simulink model "Controller"  (R2025a)
settings: Solver=ode45  StartTime=0.0  StopTime=100  RelTol=1e-5
PreLoadFcn:
  | [aircraft, state] = astSkyHogg();
undefined symbols (not defined in the file): aircraft, getCoefficient, state
libraries: aerolibasang x3, slpidlib x2, aerolibfltsims x2, shared3dof x1, sharedtransform x1
settings Model: Creator=Likith  LastModifiedBy=Likith
settings SolverCC: AlgebraicLoopSolver=TrustRegion  MinimalZcImpactIntegration=on  MaxZcPerStep=1.0
settings DataIOCC: SaveFormat=Array
settings OptimizationCC: EnhancedBackFolding=on  StrengthReduction=on  InitFltsAndDblsToZero=on  DifferentSizesBufferReuse=on
settings DebuggingCC: WriteAfterWriteMsg=DisableAll  AlgebraicLoopMsg=none  FcnCallInpInsideContextMsg=warning  UniqueDataStoreMsg=error  RootOutportRequireBusObject=none  StateNameClashWarn=warning  StrictBusMsg=ErrorOnBusTreatedAsVector  SFUnexpectedBacktrackingDiag=warning  SFNoUnconditionalDefaultTransitionDiag=warning  SFExecutionAtInitializationDiag=none  ArithmeticOperatorsInVariantConditions=warning
settings ModelReferenceCC: EnableRefExpFcnMdlSchedulingChecks=on  PropagateSignalLabelsOutOfModel=off
settings SFSimCC: SimUseLocalCustomCode=off
settings RTWCC: RTWUseLocalCustomCode=off  GPUComputeCapability=3.5  DLArmComputeVersion=19.05
settings CodeAppCC: StateflowObjectComments=on

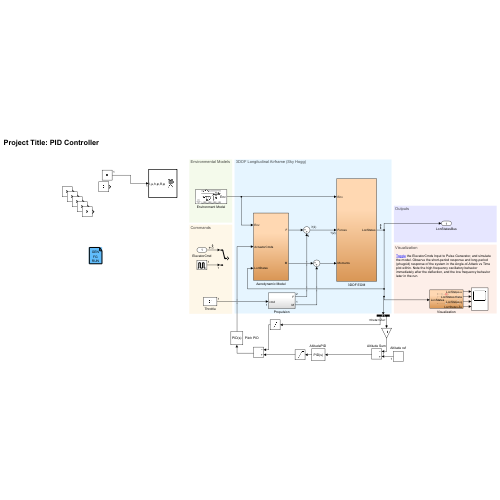
[thumbnail: Simulink's stored preview of the top-level diagram]
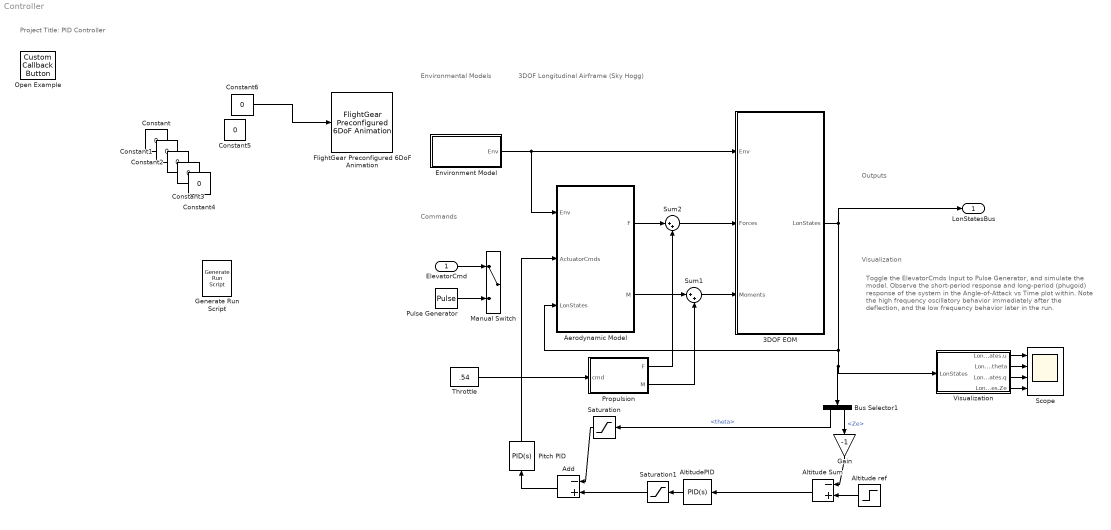
== system Controller ==
  note: Project Title: PID Controller
  note: 3DOF Longitudinal Airframe (Sky Hogg)
  note: Environmental Models
  note: Commands
  note: Toggle the ElevatorCmds Input to Pulse Generator, and simulate the model. Observe the short-period response and long-period (phugoid) response of the system in the Angle-of-Attack vs Time plot within. Note the high frequency oscillatory behavior immediately after the deflection, and the low frequency behavior later in the run.
  note: Visualization
  note: Outputs
  ElevatorCmd : Inport
  3DOF EOM : Subsystem  VariantControl=eom3DOF
  Add : Sum  Inputs=-+
  Aerodynamic Model : Subsystem  VariantControl=aeroCONST
  Altitude Sum : Sum  Inputs=-+
  Altitude ref : Step  Time=5  Before=2000  After=2200  SampleTime=0
  "AltitudePID " : slpidlib/PID Controller  Controller=PID  Form=Parallel  TimeDomain=Continuous-time  UseExternalTs=off  SampleTime=-1  IntegratorMethod=Forward Euler  FilterMethod=Forward Euler  ControllerParametersSource=internal  P=.05  I=.005  UseKiTs=off  D=0  UseExternalDerivativeSource=off  N=100  UseFilter=on  TunerSelectOption=Transfer Function Based (PID Tuner App)  InitialConditionSource=internal  InitialConditionForIntegrator=0  InitialConditionForFilter=0  DifferentiatorICPrevScaledInput=0  ExternalReset=none  TrackingMode=off  Kt=1  LimitOutput=off  SatLimitsSource=internal  UpperSaturationLimit=inf  LowerSaturationLimit=-inf  LinearizeAsGain=on  AntiWindupMode=none  Kb=1  LimitIntegrator=off  UpperIntegratorSaturationLimit=inf  LowerIntegratorSaturationLimit=-inf  POutMin=[]  POutMax=[]  IOutMin=[]  IOutMax=[]  DOutMin=[]  DOutMax=[]  NOutMin=[]  NOutMax=[]  SumOutMin=[]  SumOutMax=[]  SaturationOutMin=[]  SaturationOutMax=[]  PParamMin=[]  PParamMax=[]  IParamMin=[]  IParamMax=[]  DParamMin=[]  DParamMax=[]  NParamMin=[]  NParamMax=[]  KbParamMin=[]  KbParamMax=[]  KtParamMin=[]  KtParamMax=[]  KbOutMin=[]  KbOutMax=[]  KtOutMin=[]  KtOutMax=[]  IntegratorOutMin=[]  IntegratorOutMax=[]  FilterOutMin=[]  FilterOutMax=[]  SumI1OutMin=[]  SumI1OutMax=[]  SumI2OutMin=[]  SumI2OutMax=[]  SumI3OutMin=[]  SumI3OutMax=[]  SumI4OutMin=[]  SumI4OutMax=[]  SumDOutMin=[]  SumDOutMax=[]  DifferentiatorOutMin=[]  DifferentiatorOutMax=[]  FilterDiffOutCoefMin=[]  FilterDiffOutCoefMax=[]  ReciprocalOutMin=[]  ReciprocalOutMax=[]  SumDenOutMin=[]  SumDenOutMax=[]  SumNumOutMin=[]  SumNumOutMax=[]  DivideOutMin=[]  DivideOutMax=[]  UdiffTsProdOutMin=[]  UdiffTsProdOutMax=[]  NTsProdOutMin=[]  NTsProdOutMax=[]  UintegralTsProdOutMin=[]  UintegralTsProdOutMax=[]  UngainTsProdOutMin=[]  UngainTsProdOutMax=[]  ClampingZeroOutDataTypeStr=Inherit: Inherit via back propagation  ClampingZeroOutMin=[]  ClampingZeroOutMax=[]  FilterDenConstantOutDataTypeStr=Inherit: Inherit via back propagation  FilterDenConstantOutMin=[]  FilterDenConstantOutMax=[]  PCopyOutDataTypeStr=Inherit: Inherit via back propagation  PCopyOutMin=[]  PCopyOutMax=[]  NCopyOutDataTypeStr=Inherit: Inherit via back propagation  NCopyOutMin=[]  NCopyOutMax=[]  IntegratorContinuousStateAttributes=''  IntegratorStateMustResolveToSignalObject=off  IntegratorRTWStateStorageClass=Auto  FilterContinuousStateAttributes=''  FilterStateMustResolveToSignalObject=off  FilterRTWStateStorageClass=Auto  ParallelPVariant=InternalParameters  IdealPVariant=Disabled  IVariant=InternalParameters  DVariant=InternalParameters  IntegratorVariant=Continuous  SatVariant=Disabled  AWVariant=Passthrough  PCopyVariant=Disabled  TRVariant=Disabled  FdbkBlocksVariant=Forward  IdealPFdbkVariant=Disabled  SatFdbkVariant=Disabled  DerivativeFilterVariant=ContFilter  NVariant=InternalParameters  NCopyVariant=Disabled  FilterICVariant=InternalICsFilter  IntegratorICVariant=InternalICs  ExternalResetVariant=Disabled  TRSumVariant=Passthrough  SumFdbkVariant=Disabled  SumVariant=Sum_PID  TsampFilterVariant=InternalTs  TsampNgainVariant=Passthrough  TsampIntegralVariant=Disabled_SignalSpec  ExternalSaturationOutDataTypeStr=Inherit: Same as second input  DerivativeSourceVariant=ErrorSignal  PreIntVariant=InternalPreInt
  Bus Selector1 : BusSelector  OutputSignals=theta,Ze
  Constant{,1..6} (7 alike) : Constant  Value=0
  Environment Model : Subsystem  mask(Constant Environment Model){To=state.Environment.Temperature, a=state.Environment.SpeedOfSound, Po=state.Environment.Pressure, AirDensity=state.Environment.Density, ugvgwg=state.Environment.WindVelocity, pgqgrg=[0,0,0], g=[0;0;state.Environment.Gravity]}
      mask prompts: To "Constant Temperature (K):"; a "Constant Speed of Sound (m/s):"; Po "Constant Pressure (Pa):"; AirDensity "Constant Air Density (kg/m^3):"; ugvgwg "Constant Wind Velocity [ug vg wg] (m/s):"; pgqgrg "Constant Wind Angular Rates [pg qg rg] (rad/s):"; g "Constant Gravitational Acceleration (m/s^2):"
      mask Help: helpview(fullfile(docroot,'toolbox','aeroblks','aeroblks.map'), 'environment1');
      mask TypeOptions To: Constant Atmosphere/To
      mask TypeOptions a: Constant Atmosphere/a
      mask TypeOptions Po: Constant Atmosphere/Po
      mask TypeOptions AirDensity: Constant Atmosphere/AirDensity
      mask TypeOptions ugvgwg: Constant Wind/ugvgwg
      mask TypeOptions pgqgrg: Constant Wind/pgqgrg
      mask TypeOptions g: Constant Gravity/g
      mask DialogControl Container4 Prompt: Atmospheric Model
      mask DialogControl Container6 Prompt: Wind Model
      mask DialogControl Container8 Prompt: Gravity Model
      mask Display:
      | image('aeroenvironment.bmp','center')
      | port_label('output',1,'Env')
  FlightGear Preconfigured 6DoF Animation : aerolibfltsims/FlightGear Preconfigured 6DoF Animation  xFlightGearVersion=v2019.1  DestinationIpAddress=127.0.0.1  DestinationPort=5502  SampleTime=1/30  packetVersion=24
  Gain : Gain  Gain=-1
  Generate Run Script : aerolibfltsims/Generate Run Script  Architecture=Default  dataFlow=Send  GeometryModelName=HL20  AirportId=KSFO  RunwayId=10L  InitialAltitude=7224  InitialHeading=113  OffsetDistance=4.72  OffsetAzimuth=0  InstallScenery=off  DisableShaders=off  OriginAddress=127.0.0.1  DestinationPort=5502  OriginPort=5505  LocalAddress=127.0.0.1  OutputFileName=runfg.bat  FlightGearBaseDirectory=C:\Program Files\FlightGear
  Manual Switch : ManualSwitch
  Open Example : CustomCallbackButton  Configuration="{\"components\":[{\"name\":\"BackgroundImageComponent\",\"settings\":{\"image\":{\"size\":[0,0],\"src\":\"default\",\"srcOrientation\":\"Right\"},\"position\":[0,0,1,1]}},{\"name\":\"ButtonStateComponent\",\"settings\":{\"buttonType\":\"momentary\",\"clickFcn\":\"showExample('aeroblks\\/LongitudinalFlyingQuality3DOFAnalysisExample')\",\"onValue\":1,\"position\":[0,0,1,1],\"pressDelay\":\"500\",\"pressFcn\":\"\",\"repeatInterval\":\"0\",\"states\":[{\"horizontalAlignment\":\"center\",\"image\":{\"position\":[0,0,1,1],\"size\":[1,1],\"src\":\"default\",\"srcOrientation\":\"Right\"},\"label\":{\"color\":[0.01176470588,0.01176470588,0.01176470588,1],\"icon\":{\"size\":[0,0],\"src\":\"default\",\"srcOrientation\":\"Right\"},\"iconPlacement\":\"left\",\"opacity\":1,\"show\":true,\"text\":{\"content\":\"?\",\"font\":\"Helvetica\"}},\"labelOffset\":[0,0],\"verticalAlignment\":\"middle\"},{\"horizontalAlignment\":\"center\",\"image\":{\"position\":[0,0,1,1],\"size\":[1,1],\"src\":\"default\",\"srcOrientation\":\"Right\"},\"label\":{\"color\":[0.01176470588,0.01176470588,0.01176470588,1],\"icon\":{\"size\":[0,0],\"src\":\"default\",\"srcOrientation\":\"Right\"},\"iconPlacement\":\"left\",\"opacity\":1,\"show\":true,\"text\":{\"content\":\"?\",\"font\":\"Helvetica\"}},\"labelOffset\":[0,0],\"verticalAlignment\":\"middle\"},{\"horizontalAlignment\":\"center\",\"image\":{\"position\":[0,0,1,1],\"size\":[1,1],\"src\":\"default\",\"srcOrientation\":\"Right\"},\"label\":{\"color\":[0.01176470588,0.01176470588,0.01176470588,1],\"icon\":{\"size\":[0,0],\"src\":\"default\",\"srcOrientation\":\"Right\"},\"iconPlacement\":\"left\",\"opacity\":1,\"show\":true,\"text\":{\"content\":\"?\",\"font\":\"Helvetica\"}},\"labelOffset\":[0,0],\"verticalAlignment\":\"middle\"},{\"horizontalAlignment\":\"center\",\"image\":{\"position\":[0,0,1,1],\"size\":[1,1],\"src\":\"default\",\"srcOrientation\":\"Right\"},\"label\":{\"color\":[0.01176470588,0.01176470588,0.01176470588,1],\"icon\":{\"size\":[0,0],\"src\":\"default\",\"srcOrientation\":\"Right\"},\"iconPlacement\":\"left\",\"opacity\":1,\"show\":true,\"text\":{\"content\":\"?\",\"font\":\"Helvetica\"}},\"labelOffset\":[0,0],\"verticalAlignment\":\"middle\"}]}},{\"name\":\"ForegroundImageComponent\",\"settings\":{\"image\":{\"size\":[0,0],\"src\":\"default\",\"srcOrientation\":\"Right\"},\"isForeground\":1,\"position\":[0,0,1,1]}}],\"derived\":{\"blockParameters\":{\"AutoActivate\":true,\"ButtonText\":\"?\",\"ButtonType\":\"Momentary\",\"ClickFcn\":\"showExample('aeroblks\\/LongitudinalFlyingQuality3DOFAnalysisExample')\",\"OnValue\":1,\"PressDelay\":\"500\",\"PressFcn\":\"\",\"RepeatInterval\":\"0\",\"fixedAspectRatio\":\"off\"}},\"settings\":{\"BindingType\":\"standalone\",\"autoActivate\":true,\"backgroundColor\":[244,244,244,1],\"backgroundOffset\":0,\"backgroundOpacity\":1,\"fixedAspectRatio\":\"off\",\"foregroundColor\":[0.01176470588,0.01176470588,0.01176470588,1],\"migratedFromLegacy\":true,\"useBackgroundColor\":true,\"variant\":\"callback\",\"version\":\"R2025a\"},\"type\":\"Button\"}"  CustomBackgroundColor="{\"color\":[0.9568627451,0.9568627451,0.9568627451],\"show\":true}"
  "Pitch PID " : slpidlib/PID Controller  Controller=PID  Form=Parallel  TimeDomain=Continuous-time  UseExternalTs=off  SampleTime=-1  IntegratorMethod=Forward Euler  FilterMethod=Forward Euler  ControllerParametersSource=internal  P=-0.0316348527351476  I=-3.69110962756831e-05  UseKiTs=off  D=-6.02414839381738  UseExternalDerivativeSource=off  N=22.8565595208321  UseFilter=on  TunerSelectOption=Transfer Function Based (PID Tuner App)  InitialConditionSource=internal  InitialConditionForIntegrator=0  InitialConditionForFilter=0  DifferentiatorICPrevScaledInput=0  ExternalReset=none  TrackingMode=off  Kt=1  LimitOutput=off  SatLimitsSource=internal  UpperSaturationLimit=.35  LowerSaturationLimit=-.35  LinearizeAsGain=on  AntiWindupMode=back-calculation  Kb=1  LimitIntegrator=off  UpperIntegratorSaturationLimit=inf  LowerIntegratorSaturationLimit=-inf  POutMin=[]  POutMax=[]  IOutMin=[]  IOutMax=[]  DOutMin=[]  DOutMax=[]  NOutMin=[]  NOutMax=[]  SumOutMin=[]  SumOutMax=[]  SaturationOutMin=[]  SaturationOutMax=[]  PParamMin=[]  PParamMax=[]  IParamMin=[]  IParamMax=[]  DParamMin=[]  DParamMax=[]  NParamMin=[]  NParamMax=[]  KbParamMin=[]  KbParamMax=[]  KtParamMin=[]  KtParamMax=[]  KbOutMin=[]  KbOutMax=[]  KtOutMin=[]  KtOutMax=[]  IntegratorOutMin=[]  IntegratorOutMax=[]  FilterOutMin=[]  FilterOutMax=[]  SumI1OutMin=[]  SumI1OutMax=[]  SumI2OutMin=[]  SumI2OutMax=[]  SumI3OutMin=[]  SumI3OutMax=[]  SumI4OutMin=[]  SumI4OutMax=[]  SumDOutMin=[]  SumDOutMax=[]  DifferentiatorOutMin=[]  DifferentiatorOutMax=[]  FilterDiffOutCoefMin=[]  FilterDiffOutCoefMax=[]  ReciprocalOutMin=[]  ReciprocalOutMax=[]  SumDenOutMin=[]  SumDenOutMax=[]  SumNumOutMin=[]  SumNumOutMax=[]  DivideOutMin=[]  DivideOutMax=[]  UdiffTsProdOutMin=[]  UdiffTsProdOutMax=[]  NTsProdOutMin=[]  NTsProdOutMax=[]  UintegralTsProdOutMin=[]  UintegralTsProdOutMax=[]  UngainTsProdOutMin=[]  UngainTsProdOutMax=[]  ClampingZeroOutDataTypeStr=Inherit: Inherit via back propagation  ClampingZeroOutMin=[]  ClampingZeroOutMax=[]  FilterDenConstantOutDataTypeStr=Inherit: Inherit via back propagation  FilterDenConstantOutMin=[]  FilterDenConstantOutMax=[]  PCopyOutDataTypeStr=Inherit: Inherit via back propagation  PCopyOutMin=[]  PCopyOutMax=[]  NCopyOutDataTypeStr=Inherit: Inherit via back propagation  NCopyOutMin=[]  NCopyOutMax=[]  IntegratorContinuousStateAttributes=''  IntegratorStateMustResolveToSignalObject=off  IntegratorRTWStateStorageClass=Auto  FilterContinuousStateAttributes=''  FilterStateMustResolveToSignalObject=off  FilterRTWStateStorageClass=Auto  ParallelPVariant=InternalParameters  IdealPVariant=Disabled  IVariant=InternalParameters  DVariant=InternalParameters  IntegratorVariant=Continuous  SatVariant=Disabled  AWVariant=Passthrough  PCopyVariant=Disabled  TRVariant=Disabled  FdbkBlocksVariant=Forward  IdealPFdbkVariant=Disabled  SatFdbkVariant=Disabled  DerivativeFilterVariant=ContFilter  NVariant=InternalParameters  NCopyVariant=Disabled  FilterICVariant=InternalICsFilter  IntegratorICVariant=InternalICs  ExternalResetVariant=Disabled  TRSumVariant=Passthrough  SumFdbkVariant=Disabled  SumVariant=Sum_PID  TsampFilterVariant=InternalTs  TsampNgainVariant=Passthrough  TsampIntegralVariant=Disabled_SignalSpec  ExternalSaturationOutDataTypeStr=Inherit: Same as second input  DerivativeSourceVariant=ErrorSignal  PreIntVariant=InternalPreInt
  Propulsion : Subsystem
      settings: RTWSystemCode=Inline
  Pulse Generator : DiscretePulseGenerator  PulseType=Time based  Amplitude=-2*pi/180  Period=500  PulseWidth=.5  PhaseDelay=10
  Saturation : Saturate  UpperLimit=.5  LowerLimit=-.5
  Saturation1 : Saturate  UpperLimit=.35  LowerLimit=-.35
  Scope : Scope  NumInputPorts=4
      settings: Title=Angle of Attack vs Time  ActiveDisplayYMinimum=-0.24440307700607011  ActiveDisplayYMaximum=0.34975969790728162  YLabel=\alpha [rad]
  Sum1 : Sum  Inputs=|++  InputSameDT=on  SaturateOnIntegerOverflow=on  OutDataTypeStr=Inherit: Same as first input
  Sum2 : Sum  Inputs=|++  InputSameDT=on  SaturateOnIntegerOverflow=on  OutDataTypeStr=Inherit: Same as first input
  Throttle : Constant  Value=.54
  Visualization : Subsystem
  LonStatesBus : Outport  VectorParamsAs1DForOutWhenUnconnected=off
  wires:
  3DOF EOM/1(LonStates) -> Bus Selector1/1, Visualization/1(LonStates), Aerodynamic Model/3(LonStates), LonStatesBus/1
  Sum2/1 -> 3DOF EOM/2(Forces)
  Propulsion/2(M) -> Sum1/2
  Propulsion/1(F) -> Sum2/2
  ElevatorCmd/1 -> Manual Switch/1
  Pulse Generator/1 -> Manual Switch/2
  Throttle/1 -> Propulsion/1(cmd)
  Sum1/1 -> 3DOF EOM/3(Moments)
  Aerodynamic Model/1(F) -> Sum2/1
  Aerodynamic Model/2(" M") -> Sum1/1
  Environment Model/1(Env) -> 3DOF EOM/1(Env), Aerodynamic Model/1(Env)
  Bus Selector1/1 -> Saturation/1  "<theta>"
  Bus Selector1/2 -> Gain/1  "<Ze>"
  Altitude ref/1 -> Altitude Sum/2
  "AltitudePID "/1 -> Saturation1/1
  Visualization/1(LonStates.u) -> Scope/1
  Visualization/2(LonStates.theta) -> Scope/2
  Visualization/3(LonStates.q) -> Scope/3
  Visualization/4(LonStates.Ze) -> Scope/4
  Add/1 -> "Pitch PID "/1
  Altitude Sum/1 -> "AltitudePID "/1
  Saturation1/1 -> Add/2
  Saturation/1 -> Add/1
  "Pitch PID "/1 -> Aerodynamic Model/2(ActuatorCmds)
  Gain/1 -> Altitude Sum/1
  Constant6/1 -> FlightGear Preconfigured 6DoF Animation/1

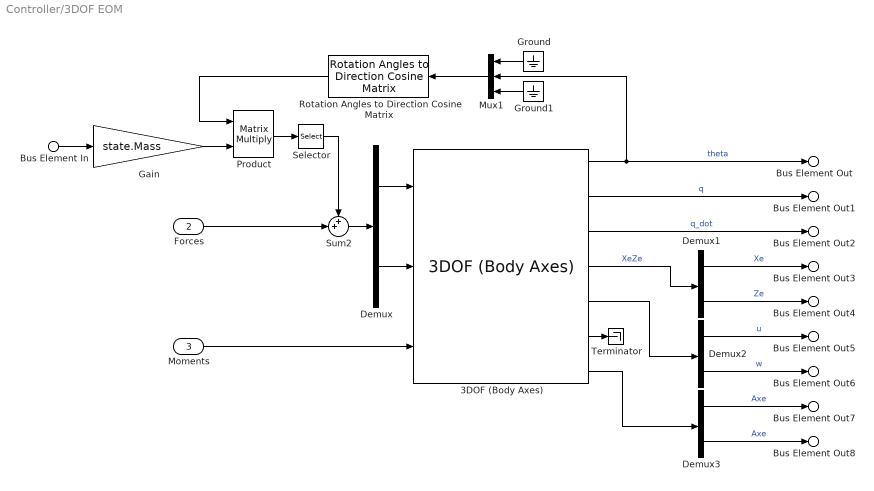
== system Controller/3DOF EOM ==
  Bus Element In : Inport  PortName=Env  Element=g
  Forces : Inport  Port=2
  Moments : Inport  Port=3
  3DOF (Body Axes) : shared3dof/3DOF (Body Axes)  units=Metric (MKS)  mtype=Fixed  v_ini=state.U  theta_ini=deg2rad(state.Theta)  alpha_ini=deg2rad(state.Alpha)  pos_ini=[state.XN, state.XD]  q_ini=state.Q  mass=state.Mass  mass_e=0.5  mass_f=3.0  Iyy=state.Inertia{2,2}  Iyy_e=0.5  Iyy_f=3.0  g_in=Internal  g=0  vre_flag=on  abi_flag=on  aMode=0  vel_statename={'u', 'w'}  theta_statename='theta'  pos_statename={'Xe', 'Ze'}  q_statename='q'  mass_statename=''
  Demux{,1..3} (4 alike) : Demux  Outputs=2
  Gain : Gain  Gain=state.Mass
  Ground : Ground
  Ground1 : Ground
  Mux1 : Mux  Inputs=3
  Product : Product  Multiplication=Matrix(*)
  Rotation Angles to Direction Cosine Matrix : sharedtransform/Rotation Angles to Direction Cosine Matrix  rotationOrder=ZYX  aMode=aMode
  Selector : Selector  InputPortWidth=3  IndexOptions=Index vector (dialog)  Indices=[1 3]  OutputSizes=1
  Sum2 : Sum  Inputs=++|  InputSameDT=on  SaturateOnIntegerOverflow=on  OutDataTypeStr=Inherit: Same as first input
  Terminator : Terminator
  Bus Element Out : Outport  VectorParamsAs1DForOutWhenUnconnected=off  PortName=LonStates  Element=theta
  Bus Element Out1 : Outport  VectorParamsAs1DForOutWhenUnconnected=off  PortName=LonStates  Element=q
  Bus Element Out2 : Outport  VectorParamsAs1DForOutWhenUnconnected=off  PortName=LonStates  Element=q_dot
  Bus Element Out3 : Outport  VectorParamsAs1DForOutWhenUnconnected=off  PortName=LonStates  Element=Xe
  Bus Element Out4 : Outport  VectorParamsAs1DForOutWhenUnconnected=off  PortName=LonStates  Element=Ze
  Bus Element Out5 : Outport  VectorParamsAs1DForOutWhenUnconnected=off  PortName=LonStates  Element=u
  Bus Element Out6 : Outport  VectorParamsAs1DForOutWhenUnconnected=off  PortName=LonStates  Element=w
  Bus Element Out7 : Outport  VectorParamsAs1DForOutWhenUnconnected=off  PortName=LonStates  Element=Axe
  Bus Element Out8 : Outport  VectorParamsAs1DForOutWhenUnconnected=off  PortName=LonStates  Element=Aze
  wires:
  Demux/2 -> 3DOF (Body Axes)/2
  Demux/1 -> 3DOF (Body Axes)/1
  Sum2/1 -> Demux/1
  Selector/1 -> Sum2/1
  Ground1/1 -> Mux1/3
  Ground/1 -> Mux1/1
  Mux1/1 -> Rotation Angles to Direction Cosine Matrix/1
  Gain/1 -> Product/2
  Rotation Angles to Direction Cosine Matrix/1 -> Product/1
  Product/1 -> Selector/1
  Forces/1 -> Sum2/2
  Bus Element In/1 -> Gain/1
  Moments/1 -> 3DOF (Body Axes)/3
  3DOF (Body Axes)/1 -> Mux1/2, Bus Element Out/1  "theta"
  3DOF (Body Axes)/2 -> Bus Element Out1/1  "q"
  3DOF (Body Axes)/3 -> Bus Element Out2/1  "q_dot"
  3DOF (Body Axes)/4 -> Demux1/1  "XeZe"
  3DOF (Body Axes)/5 -> Demux2/1
  3DOF (Body Axes)/7 -> Demux3/1
  Demux3/1 -> Bus Element Out7/1  "Axe"
  Demux3/2 -> Bus Element Out8/1  "Axe"
  Demux2/2 -> Bus Element Out6/1  "w"
  Demux2/1 -> Bus Element Out5/1  "u"
  Demux1/2 -> Bus Element Out4/1  "Ze"
  Demux1/1 -> Bus Element Out3/1  "Xe"
  3DOF (Body Axes)/6 -> Terminator/1

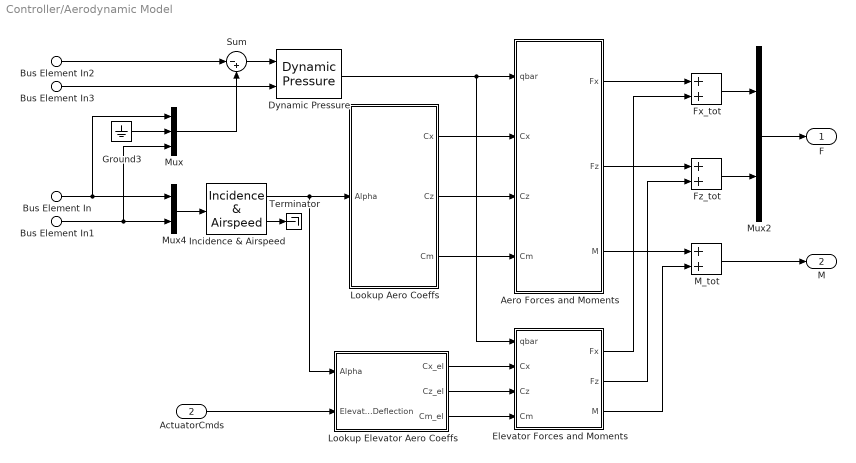
== system Controller/Aerodynamic Model ==
  Bus Element In2 : Inport  PortName=Env  Element=WindVelocity
  Bus Element In3 : Inport  PortName=Env  Element=AirDensity
  ActuatorCmds : Inport  Port=2
  Bus Element In : Inport  Port=3  PortName=LonStates  Element=u
  Bus Element In1 : Inport  Port=3  PortName=LonStates  Element=w
  Aero Forces and Moments : Subsystem
  Dynamic Pressure : aerolibasang/Dynamic Pressure
  Elevator Forces and Moments : Subsystem
  Fx_tot : Sum  InputSameDT=on  SaturateOnIntegerOverflow=on  OutDataTypeStr=Inherit: Same as first input
  Fz_tot : Sum  InputSameDT=on  SaturateOnIntegerOverflow=on  OutDataTypeStr=Inherit: Same as first input
  Ground3 : Ground
  Incidence & Airspeed : aerolibasang/Incidence  & Airspeed
  Lookup Aero Coeffs : Subsystem
  Lookup Elevator Aero Coeffs : Subsystem
  M_tot : Sum  InputSameDT=on  SaturateOnIntegerOverflow=on  OutDataTypeStr=Inherit: Same as first input
  Mux : Mux  Inputs=3
  Mux2 : Mux  Inputs=2
  Mux4 : Mux  Inputs=2
  Sum : Sum  Inputs=|-+
  Terminator : Terminator
  F : Outport  VectorParamsAs1DForOutWhenUnconnected=off
  " M" : Outport  Port=2  Unit=N*m  VectorParamsAs1DForOutWhenUnconnected=off
  wires:
  Bus Element In3/1 -> Dynamic Pressure/2
  Bus Element In2/1 -> Sum/1
  Incidence & Airspeed/2 -> Terminator/1
  Bus Element In/1 -> Mux4/1, Mux/1
  Bus Element In1/1 -> Mux4/2, Mux/3
  Mux2/1 -> F/1
  Mux4/1 -> Incidence & Airspeed/1
  Ground3/1 -> Mux/2
  M_tot/1 -> " M"/1
  ActuatorCmds/1 -> Lookup Elevator Aero Coeffs/2(Elevator Deflection)
  Sum/1 -> Dynamic Pressure/1
  Incidence & Airspeed/1 -> Lookup Elevator Aero Coeffs/1(Alpha), Lookup Aero Coeffs/1(Alpha)
  Mux/1 -> Sum/2
  Elevator Forces and Moments/3(M) -> M_tot/2
  Aero Forces and Moments/1(Fx) -> Fx_tot/1
  Aero Forces and Moments/3(M) -> M_tot/1
  Elevator Forces and Moments/1(Fx) -> Fx_tot/2
  Elevator Forces and Moments/2(Fz) -> Fz_tot/2
  Aero Forces and Moments/2(Fz) -> Fz_tot/1
  Fx_tot/1 -> Mux2/1
  Fz_tot/1 -> Mux2/2
  Lookup Elevator Aero Coeffs/1(Cx_el) -> Elevator Forces and Moments/2(Cx)
  Lookup Elevator Aero Coeffs/2(Cz_el) -> Elevator Forces and Moments/3(Cz)
  Lookup Elevator Aero Coeffs/3(Cm_el) -> Elevator Forces and Moments/4(Cm)
  Lookup Aero Coeffs/2(Cz) -> Aero Forces and Moments/3(Cz)
  Lookup Aero Coeffs/1(Cx) -> Aero Forces and Moments/2(Cx)
  Dynamic Pressure/1 -> Elevator Forces and Moments/1(qbar), Aero Forces and Moments/1(qbar)
  Lookup Aero Coeffs/3(Cm) -> Aero Forces and Moments/4(Cm)

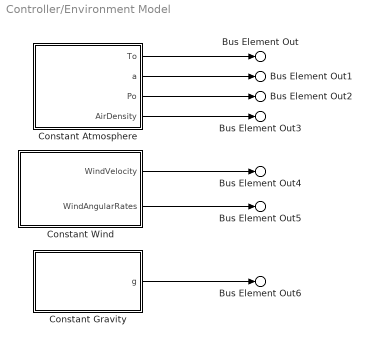
== system Controller/Environment Model ==
  Constant Atmosphere : Subsystem  VariantControl=atmosCONST  mask(Standard Atmospheric Constants){To=To, a=a, Po=Po, AirDensity=AirDensity}
      mask prompts: To "Constant Temperature (K):"; a "Constant Speed of Sound (m/s):"; Po "Constant Pressure (Pa):"; AirDensity "Constant Air Density (kg/m^3):"
  Constant Gravity : Subsystem  VariantControl=gravCONST  mask(Constant Gravitational Acceleration){g=g}
      mask prompts: g "Constant Gravitational Acceleration (m/s^2):"
  Constant Wind : Subsystem  VariantControl=windCONST  mask(Constant Wind Values){ugvgwg=ugvgwg, pgqgrg=pgqgrg}
      mask prompts: ugvgwg "Constant Wind Velocity (m/s):"; pgqgrg "Constant Wind Angular Rates (rad/s):"
  Bus Element Out : Outport  VectorParamsAs1DForOutWhenUnconnected=off  PortName=Env  Element=To
  Bus Element Out1 : Outport  VectorParamsAs1DForOutWhenUnconnected=off  PortName=Env  Element=a
  Bus Element Out2 : Outport  VectorParamsAs1DForOutWhenUnconnected=off  PortName=Env  Element=Po
  Bus Element Out3 : Outport  VectorParamsAs1DForOutWhenUnconnected=off  PortName=Env  Element=AirDensity
  Bus Element Out4 : Outport  VectorParamsAs1DForOutWhenUnconnected=off  PortName=Env  Element=WindVelocity
  Bus Element Out5 : Outport  VectorParamsAs1DForOutWhenUnconnected=off  PortName=Env  Element=WindAngularRates
  Bus Element Out6 : Outport  VectorParamsAs1DForOutWhenUnconnected=off  PortName=Env  Element=g
  wires:
  Constant Wind/2(WindAngularRates) -> Bus Element Out5/1
  Constant Atmosphere/3(Po) -> Bus Element Out2/1
  Constant Atmosphere/4(AirDensity) -> Bus Element Out3/1
  Constant Atmosphere/1(To) -> Bus Element Out/1
  Constant Wind/1(WindVelocity) -> Bus Element Out4/1
  Constant Atmosphere/2(a) -> Bus Element Out1/1
  Constant Gravity/1(g) -> Bus Element Out6/1

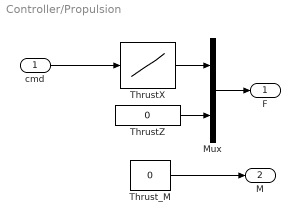
== system Controller/Propulsion ==
  cmd : Inport
  Mux : Mux  Inputs=2
  ThrustX : Lookup_n-D  NumberOfTableDimensions=1  LookupTableObject=''  BreakpointsForDimension1="getCoefficient(aircraft,\"CX\",\"Propeller\",Component=\"Propeller\").Breakpoints.Value"  IndexSearchMethod=Linear search  BeginIndexSearchUsingPreviousIndexResult=on  Table="getCoefficient(aircraft,\"CX\",\"Propeller\",Component=\"Propeller\").Table.Value"  ExtrapMethod=Clip
  ThrustZ : Constant  Value=0  SampleTime=-1
  Thrust_M : Constant  Value=0  SampleTime=-1
  F : Outport  Unit=N  VectorParamsAs1DForOutWhenUnconnected=off
  M : Outport  Port=2  Unit=N*m  VectorParamsAs1DForOutWhenUnconnected=off
  wires:
  cmd/1 -> ThrustX/1
  Thrust_M/1 -> M/1
  Mux/1 -> F/1
  ThrustZ/1 -> Mux/2
  ThrustX/1 -> Mux/1

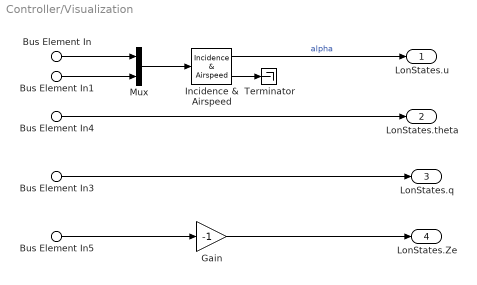
== system Controller/Visualization ==
  Bus Element In : Inport  PortName=LonStates  Element=u
  Bus Element In1 : Inport  PortName=LonStates  Element=w
  Bus Element In3 : Inport  PortName=LonStates  Element=q
  Bus Element In4 : Inport  PortName=LonStates  Element=theta
  Bus Element In5 : Inport  PortName=LonStates  Element=Ze
  Gain : Gain  Gain=-1
  Incidence & Airspeed : aerolibasang/Incidence  & Airspeed
  Mux : Mux  Inputs=2
  Terminator : Terminator
  LonStates.u : Outport  VectorParamsAs1DForOutWhenUnconnected=off
  LonStates.theta : Outport  Port=2  VectorParamsAs1DForOutWhenUnconnected=off
  LonStates.q : Outport  Port=3  VectorParamsAs1DForOutWhenUnconnected=off
  LonStates.Ze : Outport  Port=4  VectorParamsAs1DForOutWhenUnconnected=off
  wires:
  Gain/1 -> LonStates.Ze/1
  Bus Element In5/1 -> Gain/1
  Bus Element In4/1 -> LonStates.theta/1
  Bus Element In3/1 -> LonStates.q/1
  Mux/1 -> Incidence & Airspeed/1
  Bus Element In1/1 -> Mux/2
  Bus Element In/1 -> Mux/1
  Incidence & Airspeed/2 -> Terminator/1
  Incidence & Airspeed/1 -> LonStates.u/1  "alpha"

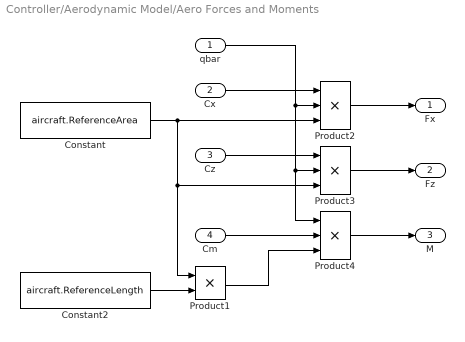
== system Controller/Aerodynamic Model/Aero Forces and Moments ==
  qbar : Inport
  Cx : Inport  Port=2
  Cz : Inport  Port=3
  Cm : Inport  Port=4
  Constant : Constant  Value=aircraft.ReferenceArea
  Constant2 : Constant  Value=aircraft.ReferenceLength
  Product1 : Product  InputSameDT=on  SaturateOnIntegerOverflow=on  OutDataTypeStr=Inherit: Same as first input
  Product2 : Product  Inputs=3  InputSameDT=on  SaturateOnIntegerOverflow=on  OutDataTypeStr=Inherit: Same as first input
  Product3 : Product  Inputs=3  InputSameDT=on  SaturateOnIntegerOverflow=on  OutDataTypeStr=Inherit: Same as first input
  Product4 : Product  Inputs=3  InputSameDT=on  SaturateOnIntegerOverflow=on  OutDataTypeStr=Inherit: Same as first input
  Fx : Outport  VectorParamsAs1DForOutWhenUnconnected=off
  Fz : Outport  Port=2  VectorParamsAs1DForOutWhenUnconnected=off
  M : Outport  Port=3  VectorParamsAs1DForOutWhenUnconnected=off
  wires:
  Cm/1 -> Product4/2
  Product3/1 -> Fz/1
  qbar/1 -> Product4/1, Product3/2, Product2/2
  Product4/1 -> M/1
  Cx/1 -> Product2/1
  Product1/1 -> Product4/3
  Product2/1 -> Fx/1
  Cz/1 -> Product3/1
  Constant/1 -> Product1/1, Product3/3, Product2/3
  Constant2/1 -> Product1/2

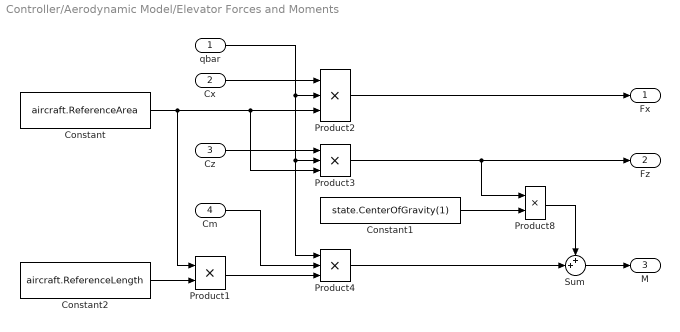
== system Controller/Aerodynamic Model/Elevator Forces and Moments ==
  qbar : Inport
  Cx : Inport  Port=2
  Cz : Inport  Port=3
  Cm : Inport  Port=4
  Constant : Constant  Value=aircraft.ReferenceArea
  Constant1 : Constant  Value=state.CenterOfGravity(1)
  Constant2 : Constant  Value=aircraft.ReferenceLength
  Product1 : Product  InputSameDT=on  SaturateOnIntegerOverflow=on  OutDataTypeStr=Inherit: Same as first input
  Product2 : Product  Inputs=3  InputSameDT=on  SaturateOnIntegerOverflow=on  OutDataTypeStr=Inherit: Same as first input
  Product3 : Product  Inputs=3  InputSameDT=on  SaturateOnIntegerOverflow=on  OutDataTypeStr=Inherit: Same as first input
  Product4 : Product  Inputs=3  InputSameDT=on  SaturateOnIntegerOverflow=on  OutDataTypeStr=Inherit: Same as first input
  Product8 : Product
  Sum : Sum  Inputs=++|
  Fx : Outport  VectorParamsAs1DForOutWhenUnconnected=off
  Fz : Outport  Port=2  VectorParamsAs1DForOutWhenUnconnected=off
  M : Outport  Port=3  VectorParamsAs1DForOutWhenUnconnected=off
  wires:
  Constant1/1 -> Product8/2
  Product1/1 -> Product4/3
  Product8/1 -> Sum/1
  Cz/1 -> Product3/1
  Cx/1 -> Product2/1
  Product4/1 -> Sum/2
  Product2/1 -> Fx/1
  Sum/1 -> M/1
  Product3/1 -> Fz/1, Product8/1
  Constant/1 -> Product1/1, Product3/3, Product2/3
  Constant2/1 -> Product1/2
  Cm/1 -> Product4/2
  qbar/1 -> Product4/1, Product3/2, Product2/2

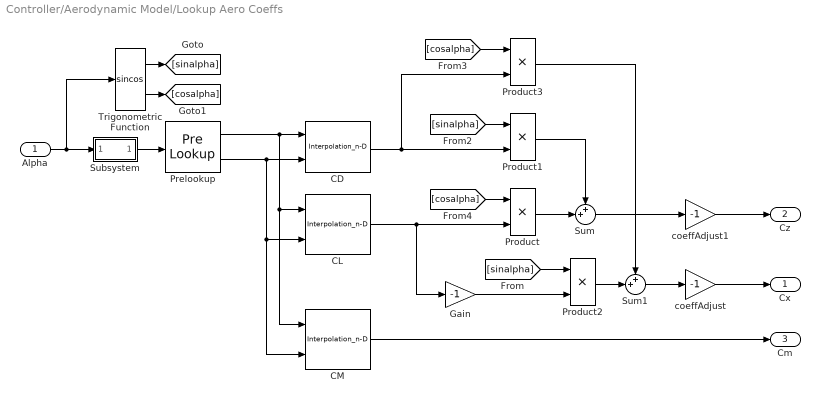
== system Controller/Aerodynamic Model/Lookup Aero Coeffs ==
  Alpha : Inport  Unit=rad
  CD : Interpolation_n-D  NumberOfTableDimensions=1  Table="getCoefficient(aircraft,\"CD\",\"Zero\").Table.Value"  InternalRulePriority=Speed
      settings: InputPortMap=u0,u1
  CL : Interpolation_n-D  NumberOfTableDimensions=1  Table="getCoefficient(aircraft,\"CL\",\"Zero\").Table.Value"  InternalRulePriority=Speed
      settings: InputPortMap=u0,u1
  CM : Interpolation_n-D  NumberOfTableDimensions=1  Table="getCoefficient(aircraft,\"Cm\",\"Zero\").Table.Value"  InternalRulePriority=Speed
      settings: InputPortMap=u0,u1
  Gain : Gain  Gain=-1
  Prelookup : PreLookup  BreakpointsData="getCoefficient(aircraft,\"CD\",\"Zero\").Breakpoints(1).Value"  ExtrapMethod=Linear
  Product{,1..3} (4 alike) : Product
  Subsystem : Subsystem
      mask Display:
      | port_label('output',1,'deg')
      | port_label('input',1,'rad')
  Sum : Sum  Inputs=++|
  Sum1 : Sum  Inputs=++|
  Trigonometric Function : Trigonometry  Operator=sincos
  coeffAdjust : Gain  Gain=-1
  coeffAdjust1 : Gain  Gain=-1
  Cx : Outport  VectorParamsAs1DForOutWhenUnconnected=off
  Cz : Outport  Port=2  VectorParamsAs1DForOutWhenUnconnected=off
  Cm : Outport  Port=3  VectorParamsAs1DForOutWhenUnconnected=off
  wires:
  CL/1 -> Gain/1, Product/2
  CM/1 -> Cm/1
  Prelookup/1 -> CM/1, CL/1, CD/1
  Prelookup/2 -> CM/2, CL/2, CD/2
  Product/1 -> Sum/2
  CD/1 -> Product3/2, Product1/2
  Product1/1 -> Sum/1
  Sum/1 -> coeffAdjust1/1
  Gain/1 -> Product2/2
  Product2/1 -> Sum1/2
  Product3/1 -> Sum1/1
  Sum1/1 -> coeffAdjust/1
  coeffAdjust1/1 -> Cz/1
  coeffAdjust/1 -> Cx/1
  Alpha/1 -> Trigonometric Function/1, Subsystem/1(In1)
  [sinalpha] -> Product2/1
  [sinalpha] -> Product1/1
  [cosalpha] -> Product3/1
  [cosalpha] -> Product/1
  Trigonometric Function/2 -> [cosalpha]
  Trigonometric Function/1 -> [sinalpha]
  Subsystem/1(Out2) -> Prelookup/1

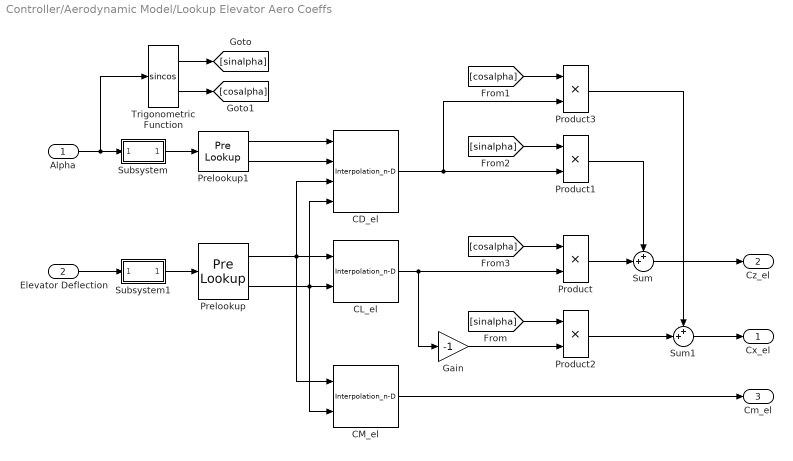
== system Controller/Aerodynamic Model/Lookup Elevator Aero Coeffs ==
  Alpha : Inport  Unit=rad
  Elevator Deflection : Inport  Port=2  Unit=rad
  CD_el : Interpolation_n-D  Table="getCoefficient(aircraft,\"CD\",\"Elevator\",Component=\"Elevator\").Table.Value"
  CL_el : Interpolation_n-D  NumberOfTableDimensions=1  Table="getCoefficient(aircraft,\"CL\",\"Elevator\",Component=\"Elevator\").Table.Value"  InternalRulePriority=Speed
      settings: InputPortMap=u0,u1
  CM_el : Interpolation_n-D  NumberOfTableDimensions=1  Table="getCoefficient(aircraft,\"Cm\",\"Elevator\",Component=\"Elevator\").Table.Value"  InternalRulePriority=Speed
      settings: InputPortMap=u0,u1
  Gain : Gain  Gain=-1
  Prelookup : PreLookup  BreakpointsData="getCoefficient(aircraft,\"CD\",\"Elevator\",Component=\"Elevator\").Breakpoints(2).Value"  ExtrapMethod=Linear  IndexDataTypeStr=int32  FractionDataTypeStr=double
  Prelookup1 : PreLookup  BreakpointsData="getCoefficient(aircraft,\"CD\",\"Elevator\",Component=\"Elevator\").Breakpoints(1).Value"  ExtrapMethod=Linear  IndexDataTypeStr=int32  FractionDataTypeStr=double
  Product{,1..3} (4 alike) : Product
  Subsystem : Subsystem
      mask Display:
      | port_label('output',1,'deg')
      | port_label('input',1,'rad')
  Subsystem1 : Subsystem
      mask Display:
      | port_label('output',1,'deg')
      | port_label('input',1,'rad')
  Sum : Sum  Inputs=++|
  Sum1 : Sum  Inputs=++|
  Trigonometric Function : Trigonometry  Operator=sincos
  Cx_el : Outport  VectorParamsAs1DForOutWhenUnconnected=off
  Cz_el : Outport  Port=2  VectorParamsAs1DForOutWhenUnconnected=off
  Cm_el : Outport  Port=3  VectorParamsAs1DForOutWhenUnconnected=off
  wires:
  Sum1/1 -> Cx_el/1
  CM_el/1 -> Cm_el/1
  Sum/1 -> Cz_el/1
  Product1/1 -> Sum/1
  Product/1 -> Sum/2
  Product2/1 -> Sum1/2
  CL_el/1 -> Product/2, Gain/1
  Product3/1 -> Sum1/1
  Gain/1 -> Product2/2
  CD_el/1 -> Product1/2, Product3/2
  Prelookup/1 -> CM_el/1, CL_el/1, CD_el/3
  Prelookup/2 -> CD_el/4, CL_el/2, CM_el/2
  Alpha/1 -> Subsystem/1(In1), Trigonometric Function/1
  Subsystem/1(Out2) -> Prelookup1/1
  Elevator Deflection/1 -> Subsystem1/1(In1)
  Prelookup1/1 -> CD_el/1
  Prelookup1/2 -> CD_el/2
  [sinalpha] -> Product2/1
  [sinalpha] -> Product1/1
  [cosalpha] -> Product3/1
  [cosalpha] -> Product/1
  Trigonometric Function/2 -> [cosalpha]
  Trigonometric Function/1 -> [sinalpha]
  Subsystem1/1(Out2) -> Prelookup/1

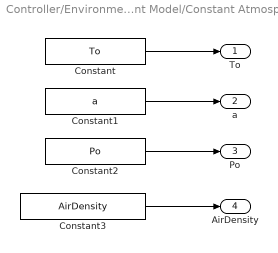
== system Controller/Environment Model/Constant Atmosphere ==
  Constant : Constant  Value=To
  Constant1 : Constant  Value=a
  Constant2 : Constant  Value=Po
  Constant3 : Constant  Value=AirDensity
  To : Outport  VectorParamsAs1DForOutWhenUnconnected=off
  a : Outport  Port=2  VectorParamsAs1DForOutWhenUnconnected=off
  Po : Outport  Port=3  VectorParamsAs1DForOutWhenUnconnected=off
  AirDensity : Outport  Port=4  VectorParamsAs1DForOutWhenUnconnected=off
  wires:
  Constant1/1 -> a/1
  Constant/1 -> To/1
  Constant2/1 -> Po/1
  Constant3/1 -> AirDensity/1

== system Controller/Environment Model/Constant Gravity ==
  Reshape1 : Reshape  OutputDimensionality=Column vector (2-D)
  Standard Gravity : Constant  Value=g
  g : Outport  VectorParamsAs1DForOutWhenUnconnected=off
  wires:
  Reshape1/1 -> g/1
  Standard Gravity/1 -> Reshape1/1

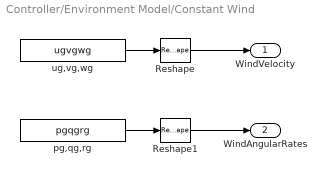
== system Controller/Environment Model/Constant Wind ==
  Reshape : Reshape  OutputDimensionality=Column vector (2-D)
  Reshape1 : Reshape  OutputDimensionality=Column vector (2-D)
  pg,qg,rg : Constant  Value=pgqgrg
  ug,vg,wg : Constant  Value=ugvgwg
  WindVelocity : Outport  VectorParamsAs1DForOutWhenUnconnected=off
  WindAngularRates : Outport  Port=2  VectorParamsAs1DForOutWhenUnconnected=off
  wires:
  pg,qg,rg/1 -> Reshape1/1
  ug,vg,wg/1 -> Reshape/1
  Reshape/1 -> WindVelocity/1
  Reshape1/1 -> WindAngularRates/1

== system Controller/Aerodynamic Model/Lookup Aero Coeffs/Subsystem ==
  In1 : Inport
  Signal Specification : SignalSpecification  Unit=deg
  Unit Conversion : UnitConversion
  Out2 : Outport  VectorParamsAs1DForOutWhenUnconnected=off
  wires:
  Signal Specification/1 -> Out2/1
  Unit Conversion/1 -> Signal Specification/1
  In1/1 -> Unit Conversion/1

== system Controller/Aerodynamic Model/Lookup Elevator Aero Coeffs/Subsystem ==
  In1 : Inport
  Signal Specification : SignalSpecification  Unit=deg
  Unit Conversion : UnitConversion
  Out2 : Outport  VectorParamsAs1DForOutWhenUnconnected=off
  wires:
  Signal Specification/1 -> Out2/1
  Unit Conversion/1 -> Signal Specification/1
  In1/1 -> Unit Conversion/1

== system Controller/Aerodynamic Model/Lookup Elevator Aero Coeffs/Subsystem1 ==
  In1 : Inport
  Signal Specification : SignalSpecification  Unit=deg
  Unit Conversion : UnitConversion
  Out2 : Outport  VectorParamsAs1DForOutWhenUnconnected=off
  wires:
  In1/1 -> Unit Conversion/1
  Unit Conversion/1 -> Signal Specification/1
  Signal Specification/1 -> Out2/1
